simulink model "progetto_metronomo1"  (R2022b)
settings: Solver=FixedStepAuto  StartTime=0.0  StopTime=100.0  FixedStep=1e-3  RelTol=1e-3
model workspace (MAT data in the model file):
  teta1 = 0
values from neighbouring files (symbols this model uses):
  k = 10    [progetto_metronomo.m]
  l = 0.1    [progetto_metronomo.m]
  m = 0.01    [progetto_metronomo.m]
  w_n = (k/m)^1/2    (= 500)    [progetto_metronomo.m]
  z = 0.1    [progetto_metronomo.m]
undefined symbols (not defined in the file or in its folder): A, A2, b, b2, g, k2, l2, m2, w_n2, z2
settings Model: Creator=huawei  LastModifiedBy=huawei

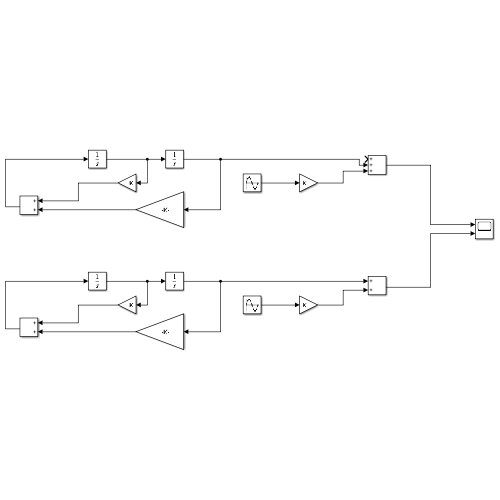
[thumbnail: Simulink's stored preview of the top-level diagram]
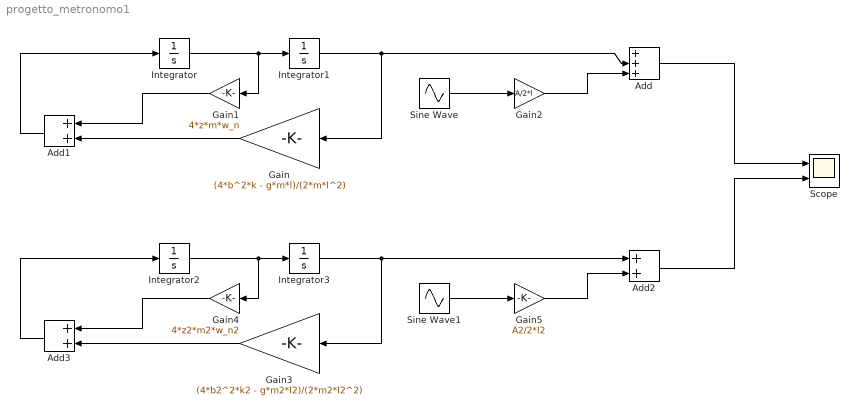
== system progetto_metronomo1 ==
  Add : Sum  Inputs=+++
  Add1 : Sum
  Add2 : Sum
  Add3 : Sum
  Gain : Gain  Gain=(4*b^2*k - g*m*l)/(2*m*l^2)
  Gain1 : Gain  Gain=4*z*m*w_n
  Gain2 : Gain  Gain=A/2*l
  Gain3 : Gain  Gain=(4*b2^2*k2 - g*m2*l2)/(2*m2*l2^2)
  Gain4 : Gain  Gain=4*z2*m2*w_n2
  Gain5 : Gain  Gain=A2/2*l2
  Integrator : Integrator
  Integrator1 : Integrator  InitialCondition=teta1
  Integrator2 : Integrator
  Integrator3 : Integrator
  Scope : Scope  NumInputPorts=2
  Sine Wave : Sin  Frequency=w_n  SampleTime=0
  Sine Wave1 : Sin  Frequency=w_n  SampleTime=0
  wires:
  Sine Wave/1 -> Gain2/1
  Gain2/1 -> Add/3
  Add/1 -> Scope/1
  Integrator1/1 -> Gain/1, Add/2
  Gain/1 -> Add1/2
  Integrator/1 -> Gain1/1, Integrator1/1
  Gain1/1 -> Add1/1
  Add1/1 -> Integrator/1
  Integrator3/1 -> Gain3/1, Add2/1
  Integrator2/1 -> Gain4/1, Integrator3/1
  Gain4/1 -> Add3/1
  Add2/1 -> Scope/2
  Gain5/1 -> Add2/2
  Sine Wave1/1 -> Gain5/1
  Gain3/1 -> Add3/2
  Add3/1 -> Integrator2/1
